simulink model "while_Sys"  (R2021a)
settings: Solver=FixedStepDiscrete  StartTime=0.0  StopTime=10.0  RelTol=1e-3
settings Model: Creator=Mohamed Elomda  LastModifiedBy=Mohamed Elomda
settings OptimizationCC: DefaultParameterBehavior=Inlined  EnhancedBackFolding=on  PassReuseOutputArgsAs=Individual arguments  ZeroExternalMemoryAtStartup=off  ZeroInternalMemoryAtStartup=off  OptimizeBlockOrder=speed  DifferentSizesBufferReuse=on  OptimizationCustomize=off  EfficientTunableParamExpr=on
settings DebuggingCC: UnderspecifiedInitializationDetection=Classic  MergeDetectMultiDrivingBlocksExec=none  ParameterTunabilityLossMsg=error
settings ModelReferenceCC: PropagateSignalLabelsOutOfModel=off
settings SFSimCC: MATLABDynamicMemAlloc=off
settings RTWCC: SystemTargetFile=ert.tlc  GenCodeOnly=on  TemplateMakefile=ert_default_tmf  GenerateReport=on  LaunchReport=on
settings CodeAppCC: ForceParamTrailComments=on  IgnoreCustomStorageClasses=off  OperatorAnnotations=on  SimulinkDataObjDesc=on  SFDataObjDesc=on  InsertBlockDesc=on
settings ERTTargetCC: TargetLangStandard=C99 (ISO)  GenerateSampleERTMain=on  InlinedParameterPlacement=NonHierarchical  ERTCustomFileTemplate=example_file_process.tlc

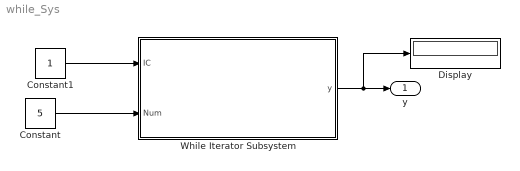
== system while_Sys ==
  Constant : Constant  Value=5  OutDataTypeStr=int32
  Constant1 : Constant  OutDataTypeStr=int32
  Display : Display
  While Iterator Subsystem : Subsystem  TreatAsAtomicUnit=on
  y : Outport
  wires:
  Constant/1 -> While Iterator Subsystem/2(Num)
  While Iterator Subsystem/1(y) -> Display/1, y/1
  Constant1/1 -> While Iterator Subsystem/1(IC)

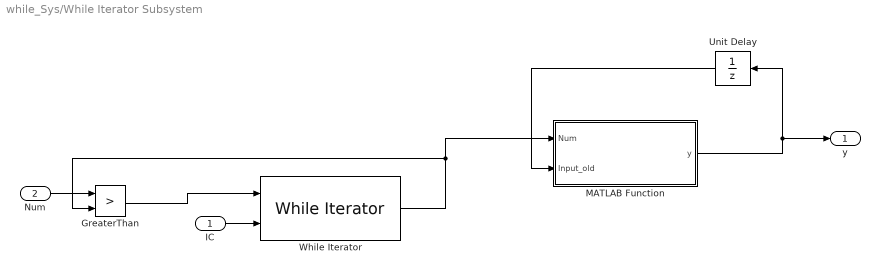
== system while_Sys/While Iterator Subsystem ==
  IC : Inport  OutDataTypeStr=int32
  Num : Inport  Port=2  OutDataTypeStr=int32
  GreaterThan : RelationalOperator  Operator=>  OutDataTypeStr=boolean  RndMeth=Simplest
  MATLAB Function : MATLAB Function  TreatAsAtomicUnit=on
  Unit Delay : UnitDelay  InitialCondition=1  SampleTime=-1  HasFrameUpgradeWarning=on
  While Iterator : WhileIterator  MaxIters=-1  ShowIterationPort=on  OutputDataType=double
  y : Outport
  wires:
  IC/1 -> While Iterator/2
  MATLAB Function/1(y) -> Unit Delay/1, y/1
  Unit Delay/1 -> MATLAB Function/2(Input_old)
  While Iterator/1 -> GreaterThan/2, MATLAB Function/1(Num)
  GreaterThan/1 -> While Iterator/1
  Num/1 -> GreaterThan/1

== matlab function while_Sys/While Iterator Subsystem/MATLAB Function ==
  data: Num input; y output; Input_old input
function y = fcn(Num,Input_old)
y = Num * Input_old;
